simulink model "InterleavingPhases"  (R2018a)
settings: Solver=FixedStepAuto  StartTime=0.0  StopTime=50  FixedStep=1e-3  RelTol=1e-3
libraries: simulink x1
settings Model: Creator=Furkan  LastModifiedBy=Furkan

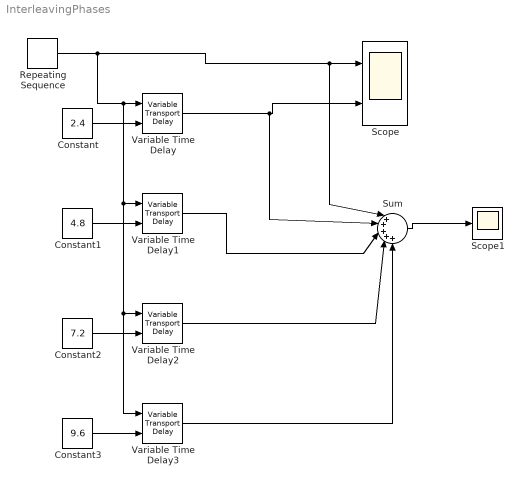
== system InterleavingPhases ==
  Constant : Constant  Value=2.4
  Constant1 : Constant  Value=4.8
  Constant2 : Constant  Value=7.2
  Constant3 : Constant  Value=9.6
  Repeating Sequence : simulink/Sources/Repeating Sequence  rep_seq_t=[0 8.1 12]  rep_seq_y=[0 1 0]
  Scope : Scope  NumInputPorts=2
  Scope1 : Scope
  Sum : Sum  Inputs=|+++++
  Variable Time Delay{,1..3} (4 alike) : VariableTransportDelay  MaximumDelay=10
  wires:
  Repeating Sequence/1 -> Variable Time Delay3/1, Variable Time Delay2/1, Variable Time Delay1/1, Variable Time Delay/1, Sum/1, Scope/1
  Constant/1 -> Variable Time Delay/2
  Variable Time Delay/1 -> Sum/2, Scope/2
  Sum/1 -> Scope1/1
  Constant1/1 -> Variable Time Delay1/2
  Variable Time Delay1/1 -> Sum/3
  Constant2/1 -> Variable Time Delay2/2
  Variable Time Delay2/1 -> Sum/4
  Constant3/1 -> Variable Time Delay3/2
  Variable Time Delay3/1 -> Sum/5
